simulink model "t_RPi_multiObj_VarS"  (R2013b)
settings: Solver=FixedStepDiscrete  StartTime=0.0  StopTime=36  RelTol=1e-3
libraries: dspsrcs4 x6, embdlinuxlib x6
settings Model: SimulationMode=external  ExtModeTrigDuration=100  Creator=mouyang  LastModifiedBy=ming
settings DataIOCC: SignalLoggingSaveFormat=ModelDataLogs
settings OptimizationCC: OptimizeModelRefInitCode=on  LifeSpan=1
settings DebuggingCC: SolverPrmCheckMsg=none  MultiTaskDSMMsg=warning  MultiTaskCondExecSysMsg=none
settings HardwareCC: ProdLargestAtomicInteger=Long  ProdLargestAtomicFloat=Double  ProdEndianess=LittleEndian  ProdHWDeviceType=ARM Compatible->ARM Cortex
settings RTWCC: SystemTargetFile=realtime.tlc  GenerateMakefile=off  TemplateMakefile=realtime.tmf  Description=Run on Target Hardware  RTWVerbose=off  ProcessScript=realtime_make_rtw_hook  IncludeERTFirstTime=on
settings STFCustomTargetCC: TargetLibSuffix=.a  GenerateSampleERTMain=on  ERTCustomFileBanners=on  SupportNonInlinedSFcns=off  SupportVariableSizeSignals=on  MATLABClassNameForMDSCustomization=Simulink.SoftwareTarget.ERTCustomization  GRTInterface=off  SystemTargetFile=realtime.tlc
settings ERTTargetCC: CodeReplacementLibrary=ANSI_C  GenerateSampleERTMain=on  ParMdlRefBuildCompliant=off  CompOptLevelCompliant=off  ConcurrentExecutionCompliant=off  CombineOutputUpdateFcns=off  ERTFirstTimeCompliant=off  SupportContinuousTime=on  SupportVariableSizeSignals=on  ModelStepFunctionPrototypeControlCompliant=off  CPPClassGenCompliant=off  ExtMode=on  ExtModeMexArgs='192.168.2.2' 0 17725  InlinedParameterPlacement=NonHierarchical  ERTSrcFileBannerTemplate=realtime_code_template.cgt  ERTHdrFileBannerTemplate=realtime_code_template.cgt  ERTDataSrcFileTemplate=realtime_code_template.cgt  ERTDataHdrFileTemplate=realtime_code_template.cgt  ERTCustomFileTemplate=realtime_file_process.tlc

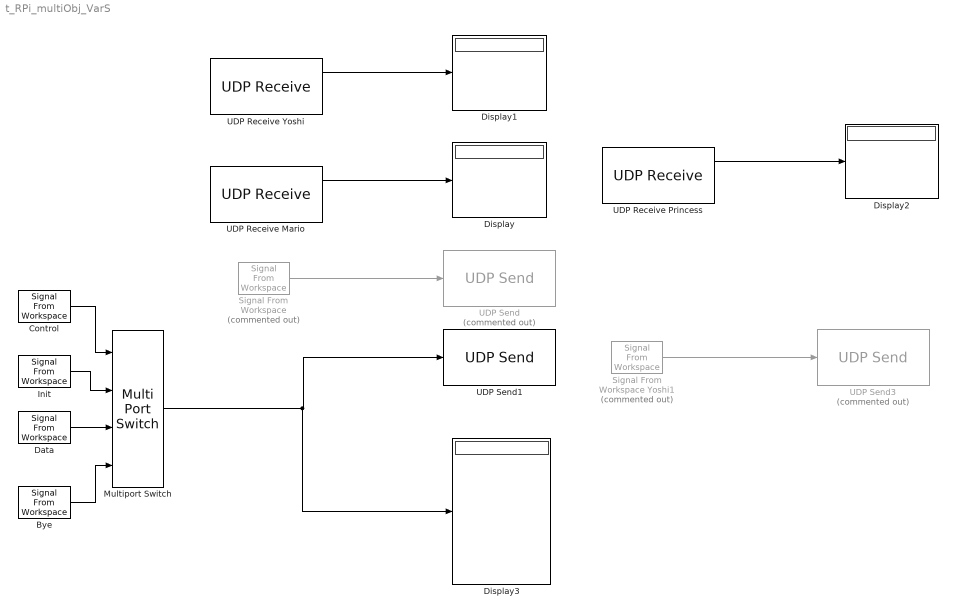
== system t_RPi_multiObj_VarS ==
  Bye : dspsrcs4/Signal From Workspace  X=uint8(200)  Ts=2  nsamps=1  OutputAfterFinalValue=Cyclic repetition  ignoreOrWarnInputAndFrameLengths=off
  Control : dspsrcs4/Signal From Workspace  X=[1 zeros(1,17)+2 3]  Ts=2  nsamps=1  OutputAfterFinalValue=Cyclic repetition  ignoreOrWarnInputAndFrameLengths=off
  Data : dspsrcs4/Signal From Workspace  X=uint8([113 1 16 123 1 13 135 1 12 113 1 0 123 1 13 133 1 16 115 1 12 123 1 0 133 1 17 113 1 23 125 1 25 113 1 16 123 1 13 135 1 12 113 1 16 123 1 13 135 1 12])  Ts=2/3  nsamps=3  OutputAfterFinalValue=Cyclic repetition  ignoreOrWarnInputAndFrameLengths=off
  Display{,1..3} (4 alike) : Display
  Init : dspsrcs4/Signal From Workspace  X=uint8([233 1 0 100 4 1])  Ts=2/6  nsamps=6  OutputAfterFinalValue=Cyclic repetition  ignoreOrWarnInputAndFrameLengths=off
  Multiport Switch : MultiPortSwitch  AllowDiffInputSizes=on
  Signal From Workspace : dspsrcs4/Signal From Workspace  Commented=on  X=uint8([213 1 0 100 4 1 113 1 16 0 0 0 113 1 13 0 0 0 115 1 12 0 0 0 213 1 0 100 4 5 113 1 16 0 0 0 113 1 13 0 0 0 115 1 12 0 0 0 213 1 0 100 4 1 113 1 16 0 0 0 113 1 13 0 0 0 115 1 12 0 0 0 200 0 0 0 0 0])  Ts=3/6  nsamps=6  OutputAfterFinalValue=Cyclic repetition  ignoreOrWarnInputAndFrameLengths=off
  Signal From Workspace Yoshi1 : dspsrcs4/Signal From Workspace  Commented=on  X=uint8([233 1 0 100 4 3 113 1 16 0 0 0 123 1 13 0 0 0 135 1 12 0 0 0 113 1 0 0 0 0 123 1 13 0 0 0 133 1 16 0 0 0 115 1 12 0 0 0 123 1 0 0 0 0 133 1 17 0 0 0 113 1 23 0 0 0 125 1 25 0 0 0 200 0 0 0 0 0])  Ts=2/6  nsamps=6  OutputAfterFinalValue=Cyclic repetition  ignoreOrWarnInputAndFrameLengths=off
  "UDP Receive Mario " : embdlinuxlib/UDP Receive  localURL='0.0.0.0'  localPort=35713  remoteURL='0.0.0.0'  remotePort=-1  recvBufferSize=8192  signalDatatype=uint8  dims=4  isVarSize=off  showBlockingTime=off  blockingTime=0  sampletime=1  blockPlatform=Raspberry Pi
  UDP Receive Princess : embdlinuxlib/UDP Receive  localURL='0.0.0.0'  localPort=35714  remoteURL='0.0.0.0'  remotePort=-1  recvBufferSize=8192  signalDatatype=uint8  dims=4  isVarSize=off  showBlockingTime=off  blockingTime=0  sampletime=1  blockPlatform=Raspberry Pi
  UDP Receive Yoshi : embdlinuxlib/UDP Receive  localURL='0.0.0.0'  localPort=35715  remoteURL='0.0.0.0'  remotePort=-1  recvBufferSize=8192  signalDatatype=uint8  dims=4  isVarSize=off  showBlockingTime=off  blockingTime=0  sampletime=1  blockPlatform=Raspberry Pi
  UDP Send : embdlinuxlib/UDP Send  Commented=on  remoteURL='127.0.0.1'  remotePort=35712  localURL='255.255.255.255'  localPortSource=Automatically determine  localPort=-1  sampletime=-1  blockPlatform=Raspberry Pi  separateLengthPort=0
  UDP Send1 : embdlinuxlib/UDP Send  remoteURL='127.0.0.1'  remotePort=35712  localURL='255.255.255.255'  localPortSource=Automatically determine  localPort=-1  sampletime=-1  blockPlatform=Raspberry Pi  separateLengthPort=0
  UDP Send3 : embdlinuxlib/UDP Send  Commented=on  remoteURL='127.0.0.1'  remotePort=35712  localURL='255.255.255.255'  localPortSource=Automatically determine  localPort=-1  sampletime=-1  blockPlatform=Raspberry Pi  separateLengthPort=0
  wires:
  "UDP Receive Mario "/1 -> Display/1
  Signal From Workspace/1 -> UDP Send/1
  UDP Receive Yoshi/1 -> Display1/1
  UDP Receive Princess/1 -> Display2/1
  Signal From Workspace Yoshi1/1 -> UDP Send3/1
  Init/1 -> Multiport Switch/2
  Bye/1 -> Multiport Switch/4
  Control/1 -> Multiport Switch/1
  Data/1 -> Multiport Switch/3
  Multiport Switch/1 -> Display3/1, UDP Send1/1
